simulink model "subsistema_hoist"  (R2023b)
settings: Solver=VariableStepAuto  StartTime=0.0  StopTime=10  RelTol=1e-3
undefined symbols (not defined in the file): bcx, bcy, bhb, bhd, bhEb, bhm, bhwu, g, h_vec, Hc, ih, J_hd_hEb, J_hm_hb, Kcy, khwu, Lh0, Ms, rhd, Thb_Max, ThEb_Max, Wc, x_LIDAR, xt_min, yh_max, yh_min, Yt0
libraries: simulink x4
settings Model: Creator=Nahuel  LastModifiedBy=rodri

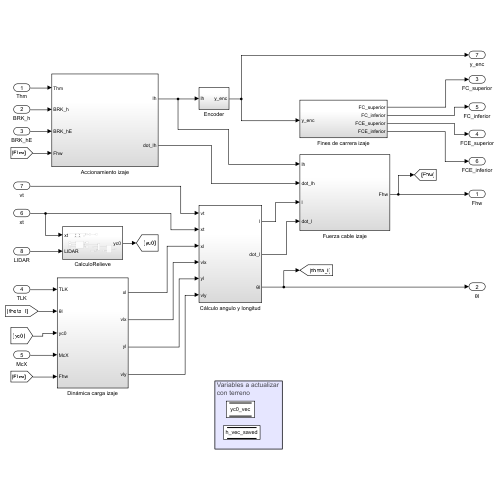
[thumbnail: Simulink's stored preview of the top-level diagram]
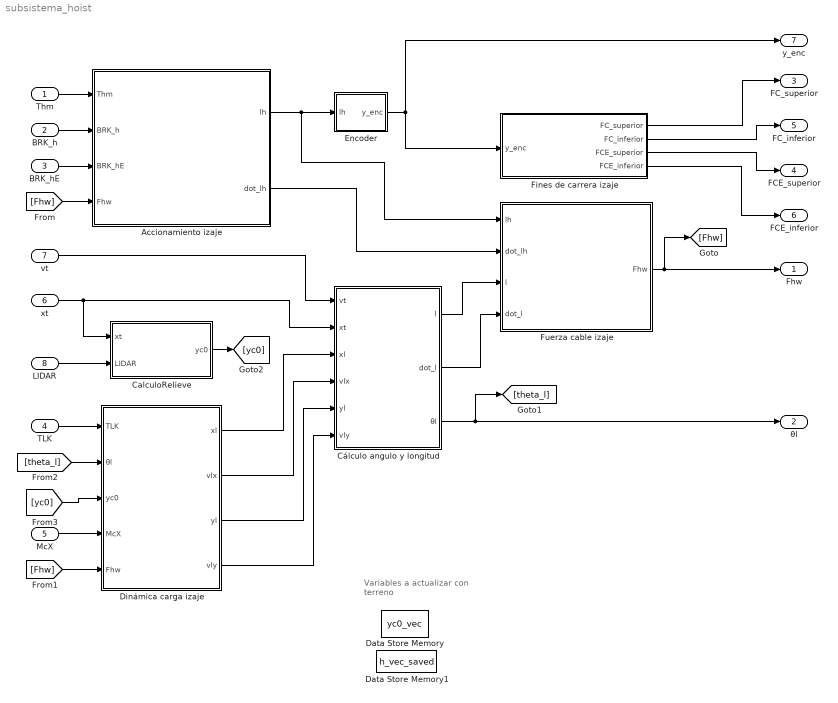
== system subsistema_hoist ==
  note: Variables a actualizar
      | con terreno
  Thm : Inport
  BRK_h : Inport  Port=2
  BRK_hE : Inport  Port=3
  TLK : Inport  Port=4
  McX : Inport  Port=5
  xt : Inport  Port=6
  vt : Inport  Port=7
  LIDAR : Inport  Port=8
  Accionamiento izaje : Subsystem
  CalculoRelieve : Subsystem
  Cálculo angulo y longitud : Subsystem
  Data Store Memory : DataStoreMemory  DataStoreName=yc0_vec  WriteAfterWriteMsg=warning  InitialValue=yc0_vec  ShowAdditionalParam=off
  Data Store Memory1 : DataStoreMemory  DataStoreName=h_vec_saved  WriteAfterWriteMsg=warning  InitialValue=h_vec_saved  ShowAdditionalParam=off
  Dinámica carga izaje : Subsystem
  Encoder : Subsystem
  Fines de carrera izaje : Subsystem
  Fuerza cable izaje : Subsystem
  Fhw : Outport
  θl : Outport  Port=2
  FC_superior : Outport  Port=3
  FCE_superior : Outport  Port=4
  FC_inferior : Outport  Port=5
  FCE_inferior : Outport  Port=6
  y_enc : Outport  Port=7
  wires:
  Thm/1 -> Accionamiento izaje/1(Thm)
  BRK_h/1 -> Accionamiento izaje/2(BRK_h)
  BRK_hE/1 -> Accionamiento izaje/3(BRK_hE)
  Accionamiento izaje/1(lh) -> Fuerza cable izaje/1(lh), Encoder/1(lh)
  Accionamiento izaje/2(dot_lh) -> Fuerza cable izaje/2(dot_lh)
  Fuerza cable izaje/1(Fhw) -> Fhw/1, [Fhw]
  [Fhw] -> Accionamiento izaje/4(Fhw)
  TLK/1 -> Dinámica carga izaje/1(TLK)
  McX/1 -> Dinámica carga izaje/4(McX)
  [Fhw] -> Dinámica carga izaje/5(Fhw)
  Dinámica carga izaje/1(xl) -> Cálculo angulo y longitud/3(xl)
  xt/1 -> CalculoRelieve/1(xt), Cálculo angulo y longitud/2(xt)
  Dinámica carga izaje/2(vlx) -> Cálculo angulo y longitud/4(vlx)
  Dinámica carga izaje/3(yl) -> Cálculo angulo y longitud/5(yl)
  Dinámica carga izaje/4(vly) -> Cálculo angulo y longitud/6(vly)
  vt/1 -> Cálculo angulo y longitud/1(vt)
  Cálculo angulo y longitud/1(l) -> Fuerza cable izaje/3(l)
  Cálculo angulo y longitud/2(dot_l) -> Fuerza cable izaje/4(dot_l)
  Cálculo angulo y longitud/3(θl) -> θl/1, [theta_l]
  [theta_l] -> Dinámica carga izaje/2(θl)
  Fines de carrera izaje/1(FC_superior) -> FC_superior/1
  Fines de carrera izaje/3(FCE_superior) -> FCE_superior/1
  Fines de carrera izaje/2(FC_inferior) -> FC_inferior/1
  Fines de carrera izaje/4(FCE_inferior) -> FCE_inferior/1
  Encoder/1(y_enc) -> y_enc/1, Fines de carrera izaje/1(y_enc)
  LIDAR/1 -> CalculoRelieve/2(LIDAR)
  CalculoRelieve/1(yc0) -> [yc0]
  [yc0] -> Dinámica carga izaje/3(yc0)

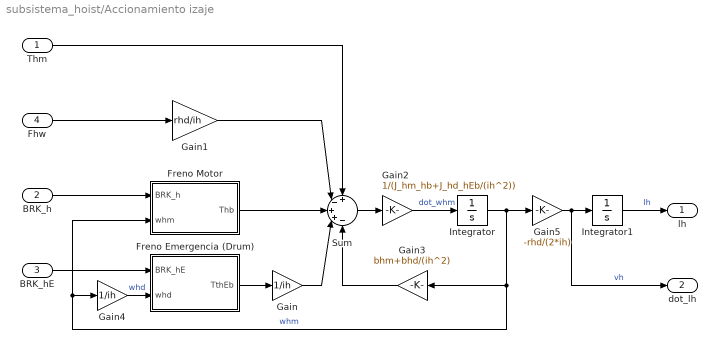
== system subsistema_hoist/Accionamiento izaje ==
  Thm : Inport
  BRK_h : Inport  Port=2
  BRK_hE : Inport  Port=3
  Fhw : Inport  Port=4
  Freno Emergencia (Drum) : Subsystem
  Freno Motor : Subsystem
  Gain : Gain  Gain=1/ih
  Gain1 : Gain  Gain=rhd/ih
  Gain2 : Gain  Gain=1/(J_hm_hb+J_hd_hEb/(ih^2))
  Gain3 : Gain  Gain=bhm+bhd/(ih^2)
  Gain4 : Gain  Gain=1/ih
  Gain5 : Gain  Gain=-rhd/(2*ih)
  Integrator : Integrator
  Integrator1 : Integrator
  Sum : Sum  Inputs=+-++-
  lh : Outport
  dot_lh : Outport  Port=2
  wires:
  Gain5/1 -> Integrator1/1, dot_lh/1  "vh"
  Integrator/1 -> Gain5/1, Gain3/1, Freno Motor/2(whm), Gain4/1  "whm"
  Freno Emergencia (Drum)/1(TthEb) -> Gain/1
  Gain3/1 -> Sum/5
  Thm/1 -> Sum/1
  BRK_h/1 -> Freno Motor/1(BRK_h)
  Gain/1 -> Sum/4
  Gain2/1 -> Integrator/1  "dot_whm"
  Sum/1 -> Gain2/1
  Gain4/1 -> Freno Emergencia (Drum)/2(whd)  "whd"
  BRK_hE/1 -> Freno Emergencia (Drum)/1(BRK_hE)
  Fhw/1 -> Gain1/1
  Freno Motor/1(Thb) -> Sum/3
  Gain1/1 -> Sum/2
  Integrator1/1 -> lh/1  "lh"

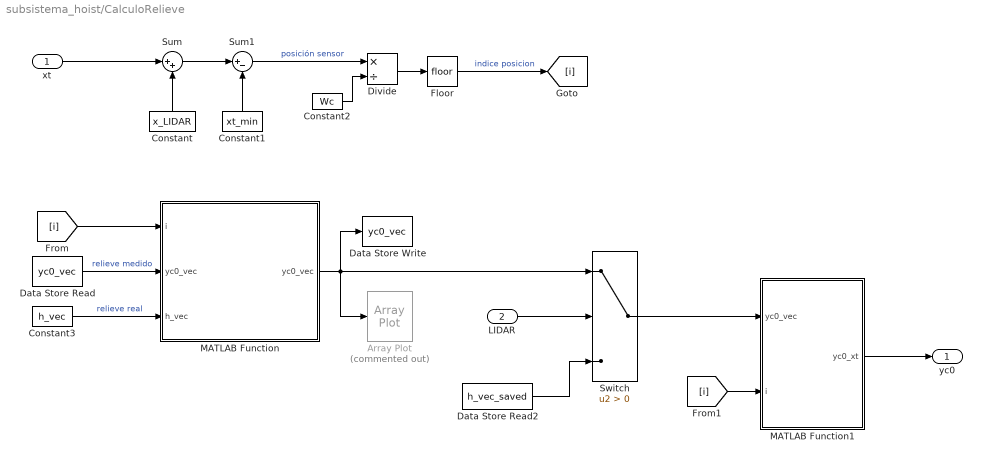
== system subsistema_hoist/CalculoRelieve ==
  xt : Inport
  LIDAR : Inport  Port=2
  Array Plot : ArrayPlot  Commented=on  WindowPosition=[563.000000,131.000000,800.000000,459.000000,]  ScopeFrameLocation=window  YLimits=[-2.5 22.5]
  Constant : Constant  Value=x_LIDAR
  Constant1 : Constant  Value=xt_min
  Constant2 : Constant  Value=Wc
  Constant3 : Constant  Value=h_vec
  Data Store Read : DataStoreRead  DataStoreName=yc0_vec  IndexOptions=Index vector (dialog)  Indices=1  OutputSizes=1
  Data Store Read2 : DataStoreRead  DataStoreName=h_vec_saved  IndexOptions=Index vector (dialog)  Indices=1  OutputSizes=1
  Data Store Write : DataStoreWrite  DataStoreName=yc0_vec  IndexOptions=Index vector (dialog)  Indices=1  OutputSizes=1
  Divide : Product  Inputs=*/
  Floor : Rounding
  MATLAB Function : MATLAB Function  TreatAsAtomicUnit=on
  MATLAB Function1 : MATLAB Function  TreatAsAtomicUnit=on
  Sum : Sum  Inputs=|++
  Sum1 : Sum  Inputs=|+-
  Switch : Switch  Criteria=u2 > Threshold  SaturateOnIntegerOverflow=off  InputSameDT=off
  yc0 : Outport
  wires:
  xt/1 -> Sum/1
  Constant/1 -> Sum/2
  Sum/1 -> Sum1/1
  Constant1/1 -> Sum1/2
  Sum1/1 -> Divide/1  "posición sensor"
  Constant2/1 -> Divide/2
  Divide/1 -> Floor/1
  Data Store Read/1 -> MATLAB Function/2("yc0_vec ")  "relieve medido"
  MATLAB Function/1(yc0_vec) -> Array Plot/1, Data Store Write/1, Switch/1
  Constant3/1 -> MATLAB Function/3(h_vec)  "relieve real"
  LIDAR/1 -> Switch/2
  Data Store Read2/1 -> Switch/3
  Switch/1 -> MATLAB Function1/1(yc0_vec)
  MATLAB Function1/1(yc0_xt) -> yc0/1
  Floor/1 -> [i]  "indice posicion"
  [i] -> MATLAB Function/1(i)
  [i] -> MATLAB Function1/2(i)

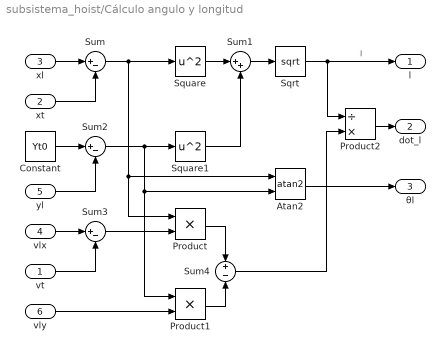
== system subsistema_hoist/Cálculo angulo y longitud ==
  vt : Inport
  xt : Inport  Port=2
  xl : Inport  Port=3
  vlx : Inport  Port=4
  yl : Inport  Port=5
  vly : Inport  Port=6
  Atan2 : Trigonometry  Operator=atan2
  Constant : Constant  Value=Yt0
  Product : Product
  Product1 : Product
  Product2 : Product  Inputs=/*
  Sqrt : Sqrt
  Square : Math  Operator=square
  Square1 : Math  Operator=square
  Sum : Sum  Inputs=|+-
  Sum1 : Sum  Inputs=|++
  Sum2 : Sum  Inputs=|+-
  Sum3 : Sum  Inputs=|+-
  Sum4 : Sum  Inputs=+-
  l : Outport
  dot_l : Outport  Port=2
  θl : Outport  Port=3
  wires:
  Product2/1 -> dot_l/1
  Sqrt/1 -> l/1, Product2/1  "l"
  Sum1/1 -> Sqrt/1
  Sum2/1 -> Product1/1, Atan2/2, Square1/1
  Sum/1 -> Product/1, Atan2/1, Square/1
  yl/1 -> Sum2/2
  Atan2/1 -> θl/1
  vly/1 -> Product1/2
  xl/1 -> Sum/1
  Constant/1 -> Sum2/1
  Sum3/1 -> Product/2
  Square1/1 -> Sum1/2
  vt/1 -> Sum3/2
  Sum4/1 -> Product2/2
  vlx/1 -> Sum3/1
  xt/1 -> Sum/2
  Square/1 -> Sum1/1
  Product1/1 -> Sum4/2
  Product/1 -> Sum4/1

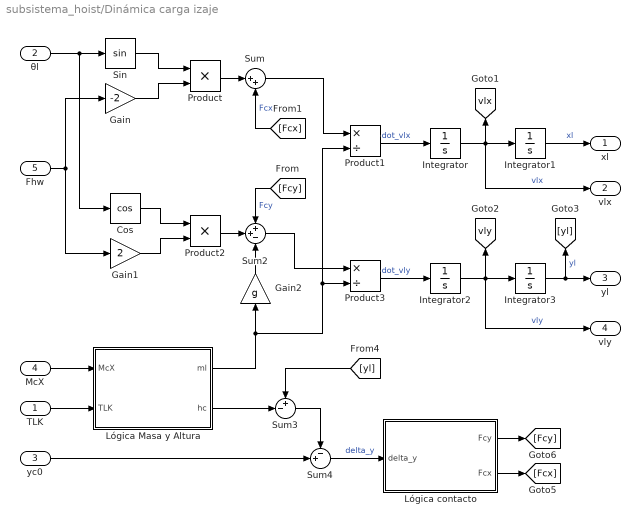
== system subsistema_hoist/Dinámica carga izaje ==
  TLK : Inport
  θl : Inport  Port=2
  yc0 : Inport  Port=3
  McX : Inport  Port=4
  Fhw : Inport  Port=5
  Cos : Trigonometry  Operator=cos
  Gain : Gain  Gain=-2
  Gain1 : Gain  Gain=2
  Gain2 : Gain  Gain=g
  Integrator{,1..3} (4 alike) : Integrator
  Lógica Masa y Altura : Subsystem
  Lógica contacto : Subsystem
  Product : Product
  Product1 : Product  Inputs=*/
  Product2 : Product
  Product3 : Product  Inputs=*/
  Sin : Trigonometry
  Sum : Sum  Inputs=|++
  Sum2 : Sum  Inputs=++-
  Sum3 : Sum  Inputs=+-|
  Sum4 : Sum  Inputs=-+|
  xl : Outport
  vlx : Outport  Port=2
  yl : Outport  Port=3
  vly : Outport  Port=4
  tag scope: vlx=global, vly=global
  wires:
  θl/1 -> Sin/1, Cos/1
  Integrator/1 -> vlx/1, Integrator1/1, [vlx]  "vlx"
  Sum3/1 -> Sum4/1
  Sin/1 -> Product/1
  Gain/1 -> Product/2
  [Fcy] -> Sum2/1  "Fcy"
  Integrator2/1 -> vly/1, Integrator3/1, [vly]  "vly"
  Integrator3/1 -> yl/1, [yl]  "yl"
  Fhw/1 -> Gain1/1, Gain/1
  [Fcx] -> Sum/2  "Fcx"
  Product/1 -> Sum/1
  Product1/1 -> Integrator/1  "dot_vlx"
  Gain2/1 -> Sum2/3
  Cos/1 -> Product2/1
  Gain1/1 -> Product2/2
  [yl] -> Sum3/1
  Product2/1 -> Sum2/2
  yc0/1 -> Sum4/2
  Sum2/1 -> Product3/1
  Product3/1 -> Integrator2/1  "dot_vly"
  Sum/1 -> Product1/1
  Integrator1/1 -> xl/1  "xl"
  Sum4/1 -> Lógica contacto/1(delta_y)  "delta_y"
  Lógica contacto/1(Fcy) -> [Fcy]
  Lógica contacto/2(Fcx) -> [Fcx]
  Lógica Masa y Altura/1(ml) -> Product1/2, Product3/2, Gain2/1
  McX/1 -> Lógica Masa y Altura/1(McX)
  TLK/1 -> Lógica Masa y Altura/2(TLK)
  Lógica Masa y Altura/2(hc) -> Sum3/2

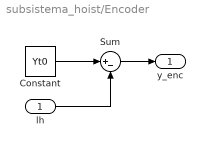
== system subsistema_hoist/Encoder ==
  lh : Inport
  Constant : Constant  Value=Yt0
  Sum : Sum  Inputs=|+-
  y_enc : Outport
  wires:
  Constant/1 -> Sum/1
  Sum/1 -> y_enc/1
  lh/1 -> Sum/2

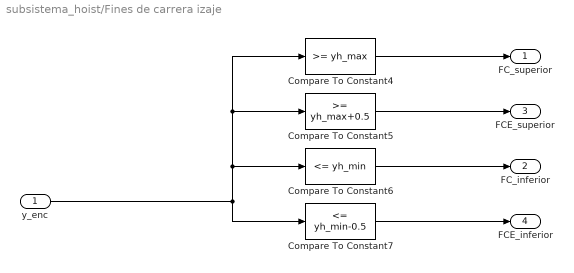
== system subsistema_hoist/Fines de carrera izaje ==
  y_enc : Inport
  Compare To Constant4 : simulink/Logic and Bit Operations/Compare To Constant  relop=>=  const=yh_max  OutDataTypeStr=boolean
  Compare To Constant5 : simulink/Logic and Bit Operations/Compare To Constant  relop=>=  const=yh_max+0.5  OutDataTypeStr=boolean
  Compare To Constant6 : simulink/Logic and Bit Operations/Compare To Constant  relop=<=  const=yh_min  OutDataTypeStr=boolean
  Compare To Constant7 : simulink/Logic and Bit Operations/Compare To Constant  relop=<=  const=yh_min-0.5  OutDataTypeStr=boolean
  FC_superior : Outport
  FC_inferior : Outport  Port=2
  FCE_superior : Outport  Port=3
  FCE_inferior : Outport  Port=4
  wires:
  Compare To Constant7/1 -> FCE_inferior/1
  y_enc/1 -> Compare To Constant4/1, Compare To Constant5/1, Compare To Constant6/1, Compare To Constant7/1
  Compare To Constant6/1 -> FC_inferior/1
  Compare To Constant5/1 -> FCE_superior/1
  Compare To Constant4/1 -> FC_superior/1

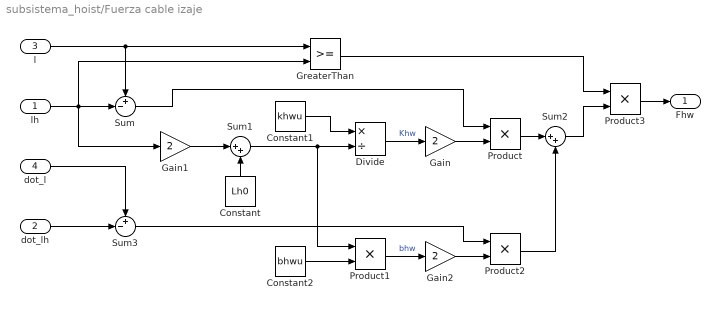
== system subsistema_hoist/Fuerza cable izaje ==
  lh : Inport
  dot_lh : Inport  Port=2
  l : Inport  Port=3
  dot_l : Inport  Port=4
  Constant : Constant  Value=Lh0
  Constant1 : Constant  Value=khwu
  Constant2 : Constant  Value=bhwu
  Divide : Product  Inputs=*/  RndMeth=Zero  SaturateOnIntegerOverflow=on
  Gain : Gain  Gain=2
  Gain1 : Gain  Gain=2
  Gain2 : Gain  Gain=2
  GreaterThan : RelationalOperator  OutDataTypeStr=boolean  RndMeth=Simplest  InputSameDT=off
  Product{,1..3} (4 alike) : Product
  Sum : Sum  Inputs=+-|
  Sum1 : Sum  Inputs=|++
  Sum2 : Sum  Inputs=|++
  Sum3 : Sum  Inputs=+-|
  Fhw : Outport
  wires:
  Constant/1 -> Sum1/2
  Constant2/1 -> Product1/2
  Sum1/1 -> Divide/2, Product1/1
  lh/1 -> Sum/2, GreaterThan/2, Gain1/1
  Product/1 -> Sum2/1
  Gain1/1 -> Sum1/1
  l/1 -> Sum/1, GreaterThan/1
  Product2/1 -> Sum2/2
  Product3/1 -> Fhw/1
  GreaterThan/1 -> Product3/1
  dot_lh/1 -> Sum3/2
  Constant1/1 -> Divide/1
  Product1/1 -> Gain2/1  "bhw"
  Sum/1 -> Product/1
  Gain2/1 -> Product2/2
  Divide/1 -> Gain/1  "Khw"
  Sum2/1 -> Product3/2
  Sum3/1 -> Product2/1
  dot_l/1 -> Sum3/1
  Gain/1 -> Product/2

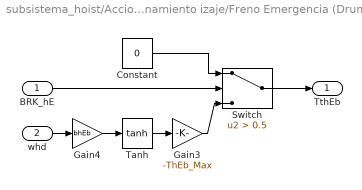
== system subsistema_hoist/Accionamiento izaje/Freno Emergencia (Drum) ==
  BRK_hE : Inport
  whd : Inport  Port=2
  Constant : Constant  Value=0
  Gain3 : Gain  Gain=-ThEb_Max
  Gain4 : Gain  Gain=bhEb
  Switch : Switch  Criteria=u2 > Threshold  Threshold=0.5  SaturateOnIntegerOverflow=off  InputSameDT=off
  Tanh : Trigonometry  Operator=tanh
  TthEb : Outport
  wires:
  BRK_hE/1 -> Switch/2
  Gain3/1 -> Switch/3
  Constant/1 -> Switch/1
  whd/1 -> Gain4/1
  Gain4/1 -> Tanh/1
  Tanh/1 -> Gain3/1
  Switch/1 -> TthEb/1

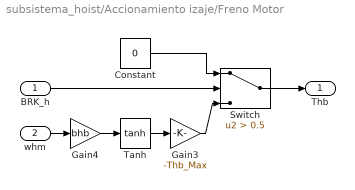
== system subsistema_hoist/Accionamiento izaje/Freno Motor ==
  BRK_h : Inport
  whm : Inport  Port=2
  Constant : Constant  Value=0
  Gain3 : Gain  Gain=-Thb_Max
  Gain4 : Gain  Gain=bhb
  Switch : Switch  Criteria=u2 > Threshold  Threshold=0.5  SaturateOnIntegerOverflow=off  InputSameDT=off
  Tanh : Trigonometry  Operator=tanh
  Thb : Outport
  wires:
  BRK_h/1 -> Switch/2
  Gain3/1 -> Switch/3
  Constant/1 -> Switch/1
  whm/1 -> Gain4/1
  Gain4/1 -> Tanh/1
  Tanh/1 -> Gain3/1
  Switch/1 -> Thb/1

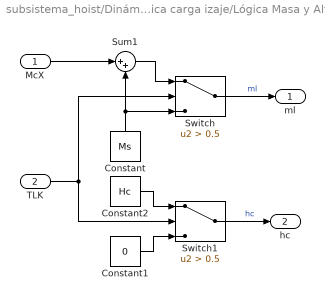
== system subsistema_hoist/Dinámica carga izaje/Lógica Masa y Altura ==
  McX : Inport
  TLK : Inport  Port=2
  Constant : Constant  Value=Ms
  Constant1 : Constant  Value=0
  Constant2 : Constant  Value=Hc
  Sum1 : Sum  Inputs=|++
  Switch : Switch  Criteria=u2 > Threshold  Threshold=0.5  SaturateOnIntegerOverflow=off  InputSameDT=off
  Switch1 : Switch  Criteria=u2 > Threshold  Threshold=0.5  SaturateOnIntegerOverflow=off  InputSameDT=off
  ml : Outport
  hc : Outport  Port=2
  wires:
  Sum1/1 -> Switch/1
  Constant2/1 -> Switch1/1
  TLK/1 -> Switch/2, Switch1/2
  Switch/1 -> ml/1  "ml"
  Constant/1 -> Switch/3, Sum1/2
  Constant1/1 -> Switch1/3
  Switch1/1 -> hc/1  "hc"
  McX/1 -> Sum1/1

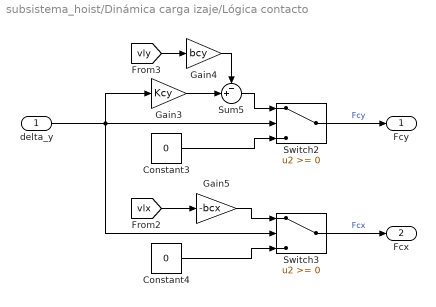
== system subsistema_hoist/Dinámica carga izaje/Lógica contacto ==
  delta_y : Inport
  Constant3 : Constant  Value=0
  Constant4 : Constant  Value=0
  Gain3 : Gain  Gain=Kcy
  Gain4 : Gain  Gain=bcy
  Gain5 : Gain  Gain=-bcx
  Sum5 : Sum  Inputs=-+|
  Switch2 : Switch  SaturateOnIntegerOverflow=off  InputSameDT=off
  Switch3 : Switch  SaturateOnIntegerOverflow=off  InputSameDT=off
  Fcy : Outport
  Fcx : Outport  Port=2
  wires:
  Sum5/1 -> Switch2/1
  [vlx] -> Gain5/1
  Gain4/1 -> Sum5/1
  [vly] -> Gain4/1
  Constant4/1 -> Switch3/3
  Gain5/1 -> Switch3/1
  Gain3/1 -> Sum5/2
  delta_y/1 -> Switch3/2, Gain3/1, Switch2/2
  Constant3/1 -> Switch2/3
  Switch2/1 -> Fcy/1  "Fcy"
  Switch3/1 -> Fcx/1  "Fcx"

== matlab function subsistema_hoist/CalculoRelieve/MATLAB Function1 ==
  data: yc0_vec input; yc0_xt output; i input
function yc0_xt = Calculo_yc0(yc0_vec,i)

yc0_xt = yc0_vec(i);

== matlab function subsistema_hoist/CalculoRelieve/MATLAB Function ==
  data: i input; yc0_vec input; yc0_vec output; h_vec input
function yc0_vec  = actualizarPerfilObstaculos(i, yc0_vec, h_vec)

if(i<=33)
    yc0_vec(i) = h_vec(i);
end
end
